simulink library "scw"  (Simulink 8.1)
settings: Solver=ode45  StartTime=0.0  StopTime=10.0  RelTol=1e-3
undefined symbols (not defined in the file or in its folder): C_TICK_TIME_S, ENUM_FCWSTATE_DBS, ENUM_FCWSTATE_DISABLED, ENUM_FCWSTATE_HAPTIC_OFF, ENUM_FCWSTATE_HAPTIC_ON, ENUM_FCWSTATE_OPERATIONAL, ENUM_FCWSTATE_PREFILL, ENUM_FCWSTATE_STANDBY, ENUM_FCWSTATE_WARNING, ENUM_HMISTATE_ACTIVE, ENUM_HMISTATE_DISABLED, ENUM_HMISTATE_STANDBY, FALSE, TRUE
settings Model: Creator=xsellart  LastModifiedBy=AT015411

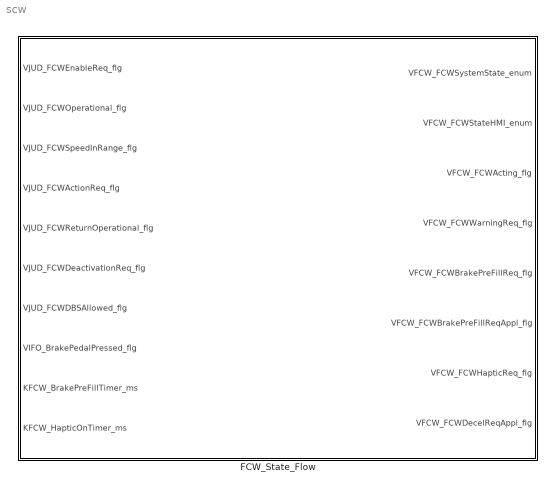
== system scw ==
  FCW_State_Flow : Stateflow chart  TreatAsAtomicUnit=on

== stateflow chart FCW_State_Flow ==
  state ENABLED
    state ACTIVE
      state OPERATIONAL
        en:
        VFCW_FCWSystemState_enum=ENUM_FCWSTATE_OPERATIONAL;
        VFCW_FCWStateHMI_enum = ENUM_HMISTATE_STANDBY;
      state ACTING
        en:
        VFCW_FCWStateHMI_enum = ENUM_HMISTATE_ACTIVE;
        VFCW_FCWActing_flg=TRUE;
        VFCW_FCWWarningReq_flg=TRUE;
        ex:
        VFCW_FCWActing_flg=FALSE;
        VFCW_FCWWarningReq_flg=FALSE;
        state WARNING
          en:
          VFCW_FCWSystemState_enum=ENUM_FCWSTATE_WARNING;
        state PREBRAKING
          VFCW_FCWBrakePreFillReq_flg = TRUE;
          VFCW_FCWBrakePreFillReqAppl_flg = TRUE;
          ex:
          VFCW_FCWBrakePreFillReq_flg = FALSE;
          VFCW_FCWBrakePreFillReqAppl_flg = FALSE;
          state HAPTIC_ON
            en:
            VFCW_FCWSystemState_enum = ENUM_FCWSTATE_HAPTIC_ON;
            VFCW_FCWHapticReq_flg = TRUE;
            VFCW_FCWDecelReqAppl_flg = TRUE;
            du:
            NFCW_MaintainTimeLocal_stp = NFCW_MaintainTimeLocal_stp + 1;
            NFCW_MaintainTimeLocal_ms = NFCW_MaintainTimeLocal_stp * C_TICK_TIME_S*1000;
            ex:
            VFCW_FCWDecelReqAppl_flg = FALSE;
            VFCW_FCWHapticReq_flg = FALSE;
            NFCW_MaintainTimeLocal_stp = 0;
            NFCW_MaintainTimeLocal_ms = 0;
          state HAPTIC_OFF
            en:
            VFCW_FCWSystemState_enum = ENUM_FCWSTATE_HAPTIC_OFF;
          state PREFILL
            en:
            VFCW_FCWSystemState_enum = ENUM_FCWSTATE_PREFILL;
            NFCW_MaintainTimeLocal_stp = 0;
            NFCW_MaintainTimeLocal_ms = 0;
            du:
            NFCW_MaintainTimeLocal_stp = NFCW_MaintainTimeLocal_stp + 1;
            NFCW_MaintainTimeLocal_ms = NFCW_MaintainTimeLocal_stp * C_TICK_TIME_S*1000;
            ex:
            NFCW_MaintainTimeLocal_stp = 0;
            NFCW_MaintainTimeLocal_ms = 0;
          (default) -> PREFILL
          HAPTIC_ON -> HAPTIC_OFF : [NFCW_MaintainTimeLocal_ms> KFCW_HapticOnTimer_ms]
          PREFILL -> HAPTIC_ON : [NFCW_MaintainTimeLocal_ms> KFCW_BrakePreFillTimer_ms]
        state BRAKE_SUPPORT
          en:
          VFCW_FCWSystemState_enum=ENUM_FCWSTATE_DBS;
          VFCW_FCWDecelReqAppl_flg = TRUE;
          ex:
          VFCW_FCWDecelReqAppl_flg = FALSE;
        (default) -> WARNING
        WARNING -> PREBRAKING : [VJUD_FCWDBSAllowed_flg==TRUE]
        PREBRAKING -> BRAKE_SUPPORT : [VIFO_BrakePedalPressed_flg==TRUE]
      (default) -> OPERATIONAL
      OPERATIONAL -> ACTING [order 2] : [VJUD_FCWActionReq_flg==TRUE]
      ACTING -> OPERATIONAL : [VJUD_FCWReturnOperational_flg==TRUE]
    state STANDBY
      en:
      VFCW_FCWSystemState_enum=ENUM_FCWSTATE_STANDBY;
      VFCW_FCWStateHMI_enum = ENUM_HMISTATE_STANDBY;
    (default) -> STANDBY
    STANDBY -> ACTIVE : [VJUD_FCWOperational_flg == TRUE]
    OPERATIONAL -> STANDBY [order 1] : [VJUD_FCWSpeedInRange_flg==FALSE]
    ACTIVE -> STANDBY : [VJUD_FCWDeactivationReq_flg==TRUE]
  state DISABLED
    en:
    VFCW_FCWSystemState_enum=ENUM_FCWSTATE_DISABLED;
    VFCW_FCWStateHMI_enum = ENUM_HMISTATE_DISABLED;
    VFCW_FCWActing_flg=FALSE;
    VFCW_FCWWarningReq_flg=FALSE;
    VFCW_FCWBrakePreFillReq_flg=FALSE;
    VFCW_FCWBrakePreFillReqAppl_flg = FALSE;
    VFCW_FCWHapticReq_flg = FALSE;
    VFCW_FCWDecelReqAppl_flg = FALSE;
  (default) -> DISABLED
  DISABLED -> ENABLED : [VJUD_FCWEnableReq_flg==TRUE]
  ENABLED -> DISABLED : [VJUD_FCWEnableReq_flg==FALSE]
  data: VJUD_FCWEnableReq_flg input double; VJUD_FCWOperational_flg input double; VJUD_FCWSpeedInRange_flg input double; VJUD_FCWActionReq_flg input double; VJUD_FCWReturnOperational_flg input double; VJUD_FCWDeactivationReq_flg input double; VJUD_FCWDBSAllowed_flg input double; VIFO_BrakePedalPressed_flg input double; VFCW_FCWSystemState_enum output uint8; ENUM_FCWSTATE_DISABLED parameter uint8 =0; ENUM_FCWSTATE_STANDBY parameter uint8 =1; ENUM_HMISTATE_ACTIVE parameter uint8 =2; ENUM_FCWSTATE_OPERATIONAL parameter uint8 =2; ENUM_FCWSTATE_WARNING parameter uint8 =3; ENUM_FCWSTATE_PREFILL parameter uint8 =4; ENUM_FCWSTATE_DBS parameter uint8 =5; VFCW_FCWStateHMI_enum output uint8; VFCW_FCWActing_flg output boolean; VFCW_FCWWarningReq_flg output boolean; VFCW_FCWBrakePreFillReq_flg output boolean; ENUM_HMISTATE_DISABLED parameter uint8; ENUM_HMISTATE_STANDBY parameter uint8; TRUE parameter boolean; FALSE parameter boolean; VFCW_FCWBrakePreFillReqAppl_flg output boolean; VFCW_FCWHapticReq_flg output boolean; VFCW_FCWDecelReqAppl_flg output boolean; ENUM_FCWSTATE_HAPTIC_ON parameter uint8; ENUM_FCWSTATE_HAPTIC_OFF parameter uint8; NFCW_MaintainTimeLocal_ms local single; NFCW_MaintainTimeLocal_stp local single; KFCW_BrakePreFillTimer_ms input single; KFCW_HapticOnTimer_ms input single; C_TICK_TIME_S parameter single
